simulink model "D53_LKA_Software"  (R2018b)
settings: Solver=ode3  StartTime=0.0  StopTime=10.0  FixedStep=0.01  RelTol=1e-3  EnableMultiTasking=on
model workspace (MAT data in the model file):
  MCOS : class17 (value not decoded)
  MCOS : class17 (value not decoded)
  MCOS : class17 (value not decoded)
  MCOS : class17 (value not decoded)
  MCOS : class17 (value not decoded)
  MCOS : class17 (value not decoded)
  MCOS : class17 (value not decoded)
  MCOS : class17 (value not decoded)
  MCOS : class17 (value not decoded)
  MCOS : class17 (value not decoded)
  MCOS : class17 (value not decoded)
  MCOS : class17 (value not decoded)
  MCOS : class17 (value not decoded)
  MCOS : class17 (value not decoded)
  MCOS : class17 (value not decoded)
  MCOS : class17 (value not decoded)
  MCOS : class17 (value not decoded)
  MCOS : class17 (value not decoded)
  MCOS : class17 (value not decoded)
  MCOS : class17 (value not decoded)
  MCOS : class17 (value not decoded)
  MCOS : class17 (value not decoded)
  MCOS : class17 (value not decoded)
  MCOS : class17 (value not decoded)
  MCOS : class17 (value not decoded)
  MCOS : class17 (value not decoded)
  MCOS : class17 (value not decoded)
  MCOS : class17 (value not decoded)
  MCOS : class17 (value not decoded)
  MCOS : class17 (value not decoded)
  MCOS : class17 (value not decoded)
  MCOS : class17 (value not decoded)
  MCOS : class17 (value not decoded)
  MCOS : class17 (value not decoded)
  MCOS : class17 (value not decoded)
  MCOS : class17 (value not decoded)
  MCOS : class17 (value not decoded)
  MCOS : class17 (value not decoded)
  MCOS : class17 (value not decoded)
  MCOS : class17 (value not decoded)
  MCOS : class17 (value not decoded)
  MCOS : class17 (value not decoded)
  MCOS : class17 (value not decoded)
  MCOS : class17 (value not decoded)
  MCOS : class17 (value not decoded)
  MCOS : class17 (value not decoded)
  MCOS : class17 (value not decoded)
  MCOS : class17 (value not decoded)
  MCOS : class17 (value not decoded)
  MCOS : class17 (value not decoded)
  MCOS : class17 (value not decoded)
  MCOS : class17 (value not decoded)
  MCOS : class17 (value not decoded)
  MCOS : class17 (value not decoded)
  MCOS : class17 (value not decoded)
  MCOS : class17 (value not decoded)
  MCOS : class17 (value not decoded)
  MCOS : class17 (value not decoded)
  MCOS : class17 (value not decoded)
  MCOS : class17 (value not decoded)
  MCOS : class17 (value not decoded)
  MCOS : class17 (value not decoded)
  MCOS : class17 (value not decoded)
  MCOS : class17 (value not decoded)
  MCOS : class17 (value not decoded)
  MCOS : class17 (value not decoded)
  MCOS : class17 (value not decoded)
  MCOS : class17 (value not decoded)
  MCOS : class17 (value not decoded)
  MCOS : class17 (value not decoded)
  MCOS : class17 (value not decoded)
  MCOS : class17 (value not decoded)
  MCOS : class17 (value not decoded)
  MCOS : class17 (value not decoded)
  MCOS : class17 (value not decoded)
  MCOS : class17 (value not decoded)
  MCOS : class17 (value not decoded)
  MCOS : class17 (value not decoded)
  MCOS : class17 (value not decoded)
  MCOS : class17 (value not decoded)
  MCOS : class17 (value not decoded)
  MCOS : class17 (value not decoded)
  MCOS : class17 (value not decoded)
  MCOS : class17 (value not decoded)
  MCOS : class17 (value not decoded)
  MCOS : class17 (value not decoded)
  MCOS : class17 (value not decoded)
  MCOS : class17 (value not decoded)
  MCOS : class17 (value not decoded)
undefined symbols (not defined in the file or in its folder): LKA_CarWidth, LKA_SampleTime, LKA_StrRatio_C, LKA_Veh2CamL_C, LKA_Veh2CamW_C, LKA_WhlBaseL_C, LL_CompSWA_C, LL_CrvtPrvwT_C, LL_DesDvt_C, LL_DvtComp_C, LL_DvtPrvwT_C, LL_DvtSpdDet_vDvtSpdMin_C, LL_HdAgExT_C, LL_HdAgPrvwT_C, LL_LAccMax_C, LL_LAccRMax_C, LL_LDW_EarliestWarnLine_C, LL_LDW_LatestWarnLine_C, LL_LDWS_SUPPRESS_HEADING, LL_LFClb_TFC_DiffCtlBalance, LL_LFClb_TFC_DiffCtrlMaxSWA, LL_LFClb_TFC_DiffCtrlRatio, LL_LFClb_TFC_facmGainLutGain1_C, LL_LFClb_TFC_facmGainLutGain2_C, LL_LFClb_TFC_facmIntegRatio, LL_LFClb_TFC_facmKlat_C, LL_LFClb_TFC_FfCtlRatio_C, LL_LFClb_TFC_phiIntegCtlMaxSWA_C, LL_LFClb_TFC_tiKlatPrvwT_C, LL_LFClb_TFC_vGainLutVehSpdLwr_C, LL_LFClb_TFC_vGainLutVehSpdUpr_C, LL_LKA_EarliestWarnLine_C, LL_LKA_LatestWarnLine_C, LL_LKAExPrcs_ExitC0Dvt, LL_LKAExPrcs_ExitC0Swt, LL_LKAExPrcs_tiExitTime1, LL_LKAExPrcs_tiExitTime2, LL_LKAExPrcs_tiExitTime3, LL_LKAS_OUT_OF_CONTROL_LAT_VEL, LL_LKAS_OUT_OF_CONTROL_TTLC, LL_LKASWASyn_M0, LL_LKASWASyn_M1, LL_LKASWASyn_M2, LL_LKASWASyn_M3K, LL_LKASWASyn_SWAaddMax, LL_LKASWASyn_T2, LL_LKASWASyn_tiTrqSwaRtTime, LL_LKASWASyn_tiTrqSwaTime, LL_LKASWASyn_TrqMax, LL_LKASWASyn_TrqSwaAddSwt, LL_LKASWASyn_TrqSwaRateDiff, LL_LSpdCompT_C, LL_lStpLngth_C, LL_MAX_DELAY_EPSSTAR_TIME, LL_MAX_DRIVER_TORQUE_DISABLE, LL_MAX_DRIVER_TORQUE_ENABLE, LL_MAX_LANE_WIDTH_DISABLE, LL_MAX_LANE_WIDTH_ENABLE, LL_MAX_LAT_ACC_DISABLE, LL_MAX_LAT_ACC_ENABLE ... (+30)
libraries: simulink x167, canmsglib x52, dspstat3 x3, simulink_extras x1
(part 18 of 21)

== system D53_LKA_Software/LL/LLOn/LL State Determination (LLStateDet)/LL State Machine Conditions (LLSMCon)/Disable Condition (DisblC)/Subsystem/Subsystem7 ==
  in1 : Inport
  Add : Sum
  Cast To Single : DataTypeConversion  OutDataTypeStr=uint8
  Memory : Memory  InheritSampleTime=on
  Saturation : Saturate  UpperLimit=1  LowerLimit=0
  Out1 : Outport
  wires:
  Saturation/1 -> Out1/1, Add/2
  Add/1 -> Memory/1
  Memory/1 -> Saturation/1
  in1/1 -> Cast To Single/1
  Cast To Single/1 -> Add/1

== system D53_LKA_Software/LL/LLOn/LL State Determination (LLStateDet)/LL State Machine Conditions (LLSMCon)/Disable Condition (DisblC)/Subsystem/Subsystem8 ==
  in1 : Inport
  Add : Sum
  Cast To Single : DataTypeConversion  OutDataTypeStr=uint8
  Memory : Memory  InheritSampleTime=on
  Saturation : Saturate  UpperLimit=1  LowerLimit=0
  Out1 : Outport
  wires:
  Saturation/1 -> Out1/1, Add/2
  Add/1 -> Memory/1
  Memory/1 -> Saturation/1
  in1/1 -> Cast To Single/1
  Cast To Single/1 -> Add/1

== system D53_LKA_Software/LL/LLOn/LL State Determination (LLStateDet)/LL State Machine Conditions (LLSMCon)/Disable Condition (DisblC)/Subsystem/Subsystem9 ==
  in1 : Inport
  Add : Sum
  Cast To Single : DataTypeConversion  OutDataTypeStr=uint8
  Memory : Memory  InheritSampleTime=on
  Saturation : Saturate  UpperLimit=1  LowerLimit=0
  Out1 : Outport
  wires:
  Cast To Single/1 -> Add/1
  in1/1 -> Cast To Single/1
  Memory/1 -> Saturation/1
  Add/1 -> Memory/1
  Saturation/1 -> Add/2, Out1/1

== system D53_LKA_Software/LL/LLOn/LL State Determination (LLStateDet)/LL State Machine Conditions (LLSMCon)/Disable Condition (DisblC)/Vehicle State Condition (VehStateC)/Emergency Light Enable Condition (EmgcyLghtEC) ==
  EmgcyLghtEC_bsStLampState : Inport
  Add : Sum
  Bus Selector : BusSelector  OutputSignals=BCM_Double_Light,BCM_Left_Light,BCM_Right_Light
  Compare To Constant{,1..3} (4 alike) : simulink/Logic and Bit Operations/Compare To Constant  relop=>  const=0  OutDataTypeStr=boolean
  Constant : Constant  Value=3  OutDataTypeStr=single
  Constant1 : Constant  Value=-1  OutDataTypeStr=single
  Logical Operator : Logic  Operator=OR  Inputs=3  AllPortsSameDT=off  OutDataTypeStr=boolean
  Memory : Memory  InheritSampleTime=on
  Saturation : Saturate  UpperLimit=200  LowerLimit=-1
  Switch : Switch  Criteria=u2 > Threshold
  EmgcyLghtEC_stEmgcyLghtECFlg : Outport
  wires:
  Compare To Constant2/1 -> Logical Operator/2
  Compare To Constant1/1 -> Logical Operator/1
  EmgcyLghtEC_bsStLampState/1 -> Bus Selector/1
  Bus Selector/1 -> Compare To Constant1/1  "<BCM_Double_Light>"
  Bus Selector/2 -> Compare To Constant2/1  "<BCM_Left_Light>"
  Logical Operator/1 -> Switch/2
  Constant/1 -> Switch/1
  Constant1/1 -> Switch/3
  Switch/1 -> Add/1
  Add/1 -> Saturation/1
  Saturation/1 -> Compare To Constant/1, Memory/1
  Memory/1 -> Add/2
  Compare To Constant/1 -> EmgcyLghtEC_stEmgcyLghtECFlg/1
  Bus Selector/3 -> Compare To Constant3/1  "<BCM_Right_Light>"
  Compare To Constant3/1 -> Logical Operator/3

== system D53_LKA_Software/LL/LLOn/LL State Determination (LLStateDet)/LL State Machine Conditions (LLSMCon)/Disable Condition (DisblC)/Vehicle State Condition (VehStateC)/Gear Disable Condition (GearDC) ==
  In1 : Inport
  Compare To Constant : simulink/Logic and Bit Operations/Compare To Constant  relop=~=  const=3  OutDataTypeStr=boolean
  GearDC_stGearDCFlg : Outport
  wires:
  In1/1 -> Compare To Constant/1
  Compare To Constant/1 -> GearDC_stGearDCFlg/1

== system D53_LKA_Software/LL/LLOn/LL State Determination (LLStateDet)/LL State Machine Conditions (LLSMCon)/Disable Condition (DisblC)/Vehicle State Condition (VehStateC)/Vehicle Speed Disable Condition (VehSpdDC) ==
  VehSpdDC_stDACMode : Inport
  VehSpdDC_vVehSpd : Inport  Port=2
  VehSpdDC_vLDWVehSpdMax_C : Inport  Port=3
  VehSpdDC_vLKAVehSpdMax_C : Inport  Port=4
  VehSpdDC_vVehSpdMin_C : Inport  Port=5
  Interval Test Dynamic : simulink/Logic and Bit Operations/Interval Test Dynamic  IntervalClosedRight=off  IntervalClosedLeft=off  OutDataTypeStr=boolean
      settings: SourceProductName=Simulink  SourceProductBaseCode=SL
  Logical Operator : Logic  Operator=NOT  AllPortsSameDT=off  OutDataTypeStr=boolean
  Switch : Switch  Threshold=2
  VehSpdDC_stVehSpdDCFlg : Outport
  wires:
  Interval Test Dynamic/1 -> Logical Operator/1
  VehSpdDC_vVehSpd/1 -> Interval Test Dynamic/2
  VehSpdDC_vVehSpdMin_C/1 -> Interval Test Dynamic/3
  Logical Operator/1 -> VehSpdDC_stVehSpdDCFlg/1
  VehSpdDC_stDACMode/1 -> Switch/2
  VehSpdDC_vLKAVehSpdMax_C/1 -> Switch/1
  Switch/1 -> Interval Test Dynamic/1
  VehSpdDC_vLDWVehSpdMax_C/1 -> Switch/3

== system D53_LKA_Software/LL/LLOn/LL State Determination (LLStateDet)/LL State Machine Conditions (LLSMCon)/Disable Condition (DisblC)/Vehicle State Condition (VehStateC)/Vehicle State Condition Synthesis (VehStateCSyn) ==
  VehStateCSyn_stVehSpdDCFlg : Inport
  VehStateCSyn_stEmgcyLghtDCFlg : Inport  Port=2
  VehStateCSyn_stGearDCFlg : Inport  Port=3
  Logical Operator3 : Logic  Operator=OR  Inputs=3  AllPortsSameDT=off  OutDataTypeStr=boolean
  VehStateCSyn_stVehStateCSyn : Outport
  wires:
  VehStateCSyn_stVehSpdDCFlg/1 -> Logical Operator3/1
  VehStateCSyn_stGearDCFlg/1 -> Logical Operator3/3
  Logical Operator3/1 -> VehStateCSyn_stVehStateCSyn/1
  VehStateCSyn_stEmgcyLghtDCFlg/1 -> Logical Operator3/2

== system D53_LKA_Software/LL/LLOn/LL State Determination (LLStateDet)/LL State Machine Conditions (LLSMCon)/Enable Condition (EnaC)/Enable Condition Synthesis (EnaCSyn)/If Action Subsystem ==
  Action Port : ActionPort  InitializeStates=reset
  Constant : Constant  OutDataTypeStr=boolean  SampleTime=-1
  Out : Outport
  wires:
  Constant/1 -> Out/1

== system D53_LKA_Software/LL/LLOn/LL State Determination (LLStateDet)/LL State Machine Conditions (LLSMCon)/Enable Condition (EnaC)/Enable Condition Synthesis (EnaCSyn)/If Action Subsystem2 ==
  Action Port : ActionPort  InitializeStates=reset
  Constant : Constant  OutDataTypeStr=boolean  SampleTime=-1
  Out : Outport
  wires:
  Constant/1 -> Out/1

== system D53_LKA_Software/LL/LLOn/LL State Determination (LLStateDet)/LL State Machine Conditions (LLSMCon)/Enable Condition (EnaC)/Enable Condition Synthesis (EnaCSyn)/If Action Subsystem3 ==
  Action Port : ActionPort  InitializeStates=reset
  Constant : Constant  Value=0  OutDataTypeStr=boolean
  Out : Outport
  wires:
  Constant/1 -> Out/1

== system D53_LKA_Software/LL/LLOn/LL State Determination (LLStateDet)/LL State Machine Conditions (LLSMCon)/Enable Condition (EnaC)/Enable Condition Synthesis (EnaCSyn)/If Action Subsystem4 ==
  Action Port : ActionPort  InitializeStates=reset
  Constant : Constant  Value=0  OutDataTypeStr=boolean
  Out : Outport
  wires:
  Constant/1 -> Out/1

== system D53_LKA_Software/LL/LLOn/LL State Determination (LLStateDet)/LL State Machine Conditions (LLSMCon)/Enable Condition (EnaC)/LDW Own Condition (LDWOwnC)/LDW Own Condition Synthesis (LDWOwnCSyn) ==
  LDWOwnCSyn_stDACMode : Inport
  LDWOwnCSyn_stVehPosChk : Inport  Port=2
  Compare To Constant : simulink/Logic and Bit Operations/Compare To Constant  relop=>=  const=1  OutDataTypeStr=boolean
  Compare To Constant1 : simulink/Logic and Bit Operations/Compare To Constant  relop===  const=1  OutDataTypeStr=boolean
  Logical Operator : Logic  AllPortsSameDT=off  OutDataTypeStr=boolean
  LDWOwnCSyn_stLDWOwnCSyn : Outport
  wires:
  LDWOwnCSyn_stDACMode/1 -> Compare To Constant/1
  LDWOwnCSyn_stVehPosChk/1 -> Compare To Constant1/1
  Compare To Constant/1 -> Logical Operator/1
  Compare To Constant1/1 -> Logical Operator/2
  Logical Operator/1 -> LDWOwnCSyn_stLDWOwnCSyn/1

== system D53_LKA_Software/LL/LLOn/LL State Determination (LLStateDet)/LL State Machine Conditions (LLSMCon)/Enable Condition (EnaC)/LDW Own Condition (LDWOwnC)/Vehicle Position Check (VehPosChk) ==
  VehPosChk_LaneWidth : Inport
  VehPosChk_bsDvtInfo : Inport  Port=2
  VehPosChk_lWarnLine_C : Inport  Port=3
  Bus Selector : BusSelector  OutputSignals=ILftDvt,IRgtDvt
  Logical Operator : Logic  AllPortsSameDT=off  OutDataTypeStr=boolean
  Relational Operator1 : RelationalOperator  OutDataTypeStr=boolean  RndMeth=Nearest
  Relational Operator2 : RelationalOperator  OutDataTypeStr=boolean  RndMeth=Nearest
  Subsystem : Subsystem
  VehPosChk_stVehPosChk : Outport
  wires:
  Bus Selector/1 -> Relational Operator1/1  "<ILftDvt>"
  Bus Selector/2 -> Relational Operator2/1  "<IRgtDvt>"
  Relational Operator1/1 -> Logical Operator/1
  Relational Operator2/1 -> Logical Operator/2
  Logical Operator/1 -> VehPosChk_stVehPosChk/1
  VehPosChk_bsDvtInfo/1 -> Bus Selector/1
  Subsystem/1(EnableLine) -> Relational Operator1/2, Relational Operator2/2
  VehPosChk_lWarnLine_C/1 -> Subsystem/1(WarnLine_C)
  VehPosChk_LaneWidth/1 -> Subsystem/2(LaneWidth)

== system D53_LKA_Software/LL/LLOn/LL State Determination (LLStateDet)/LL State Machine Conditions (LLSMCon)/Enable Condition (EnaC)/LKA Own Condition (LKAOwnC)/EPS State Condition (EPSStC) ==
  EPSStC_bsEPSInfo : Inport
  Bus Selector : BusSelector  OutputSignals=EPS_LKA_State
  Compare To Constant1 : simulink/Logic and Bit Operations/Compare To Constant  relop===  const=2  OutDataTypeStr=boolean
  Compare To Constant2 : simulink/Logic and Bit Operations/Compare To Constant  relop===  const=1  OutDataTypeStr=boolean
  Logical Operator : Logic  Operator=OR  AllPortsSameDT=off  OutDataTypeStr=boolean
  EPSStC_tfEPSCtlEC : Outport
  wires:
  EPSStC_bsEPSInfo/1 -> Bus Selector/1
  Logical Operator/1 -> EPSStC_tfEPSCtlEC/1
  Bus Selector/1 -> Compare To Constant2/1, Compare To Constant1/1  "<EPS_LKA_State>"
  Compare To Constant1/1 -> Logical Operator/1
  Compare To Constant2/1 -> Logical Operator/2

== system D53_LKA_Software/LL/LLOn/LL State Determination (LLStateDet)/LL State Machine Conditions (LLSMCon)/Enable Condition (EnaC)/LKA Own Condition (LKAOwnC)/Exit Lane Delay (ExLaneDel) ==
  ExLaneDel_stVehExLane : Inport
  ExLaneDel_tiExLaneDelT : Inport  Port=2
  Bus Selector2 : BusSelector  OutputSignals=LKA_SampleTime
  Cast To Single1 : DataTypeConversion  OutDataTypeStr=uint16
  Compare To Zero : simulink/Logic and Bit Operations/Compare To Zero  relop===  OutDataTypeStr=boolean
  Detect Fall Nonpositive : simulink/Logic and Bit Operations/Detect Fall Nonpositive  vinit=0  OutDataTypeStr=boolean
      settings: SourceProductName=Simulink  SourceProductBaseCode=SL
  Detect Rise Positive1 : simulink/Logic and Bit Operations/Detect Rise Positive  vinit=0  OutDataTypeStr=boolean
  Divide : Product  Inputs=*/
  If Action Subsystem3 : Subsystem  TreatAsAtomicUnit=on
  If Action Subsystem4 : Subsystem  TreatAsAtomicUnit=on
  If Action Subsystem5 : Subsystem  TreatAsAtomicUnit=on
  If1 : If  NumInputs=4  IfExpression=u1 == 1 & u2 == 1  ElseIfExpressions=u3 == 0 & u4 == 1
  Memory1 : Memory  InheritSampleTime=on
  Memory2 : Memory  InheritSampleTime=on
  Merge : Merge  Inputs=3
  Sum Condition1 : Subsystem  TreatAsAtomicUnit=on
  ExLaneDel_stExLaneDel : Outport
  wires:
  Merge/1 -> Memory1/1, Sum Condition1/1(In), Sum Condition1/Enable, Compare To Zero/1
  Memory1/1 -> If Action Subsystem5/1(In1)
  Memory2/1 -> Detect Fall Nonpositive/1, If1/3
  ExLaneDel_tiExLaneDelT/1 -> Divide/1
  If1/2 -> If Action Subsystem4/Action
  If1/1 -> If Action Subsystem3/Action
  If1/3 -> If Action Subsystem5/Action
  Detect Rise Positive1/1 -> If1/2
  ExLaneDel_stVehExLane/1 -> If1/1, Detect Rise Positive1/1
  Detect Fall Nonpositive/1 -> If1/4
  If Action Subsystem3/1(Out) -> Merge/1
  If Action Subsystem5/1(Out) -> Merge/3
  If Action Subsystem4/1(Out) -> Merge/2
  Sum Condition1/1(Out) -> Memory2/1
  Compare To Zero/1 -> ExLaneDel_stExLaneDel/1
  Divide/1 -> Cast To Single1/1
  Bus Selector2/1 -> Divide/2  "<LKA_SampleTime>"
  [LLClb_bsConstantClb] -> Bus Selector2/1
  Cast To Single1/1 -> Sum Condition1/2(Sum)

== system D53_LKA_Software/LL/LLOn/LL State Determination (LLStateDet)/LL State Machine Conditions (LLSMCon)/Enable Condition (EnaC)/LKA Own Condition (LKAOwnC)/LKA Own Condition Synthesis (LKAOwnCSyn) ==
  LKAOwnCSyn_stDACMode : Inport
  LKAOwnCSyn_stEPSCtlEC : Inport  Port=2
  LKAOwnCSyn_stVehLSpdC : Inport  Port=3
  LKAOwnCSyn_stVehPosChk : Inport  Port=4
  LKAOwnCSyn_stExLaneDel : Inport  Port=5
  Compare To Constant : simulink/Logic and Bit Operations/Compare To Constant  relop===  const=2  OutDataTypeStr=boolean
  Compare To Constant{1..2,4..5} (4 alike) : simulink/Logic and Bit Operations/Compare To Constant  relop===  const=1  OutDataTypeStr=boolean
  Logical Operator : Logic  Inputs=4  AllPortsSameDT=off  OutDataTypeStr=boolean
  LKAOwnCSyn_stLKAPptyCSyn : Outport
  wires:
  LKAOwnCSyn_stDACMode/1 -> Compare To Constant/1
  LKAOwnCSyn_stVehPosChk/1 -> Compare To Constant1/1
  Logical Operator/1 -> LKAOwnCSyn_stLKAPptyCSyn/1
  LKAOwnCSyn_stEPSCtlEC/1 -> Compare To Constant2/1
  LKAOwnCSyn_stExLaneDel/1 -> Compare To Constant5/1
  Compare To Constant/1 -> Logical Operator/1
  Compare To Constant2/1 -> Logical Operator/2
  Compare To Constant4/1 -> Logical Operator/3
  Compare To Constant1/1 -> Logical Operator/4
  Compare To Constant5/1 -> ?
  LKAOwnCSyn_stVehLSpdC/1 -> Compare To Constant4/1

== system D53_LKA_Software/LL/LLOn/LL State Determination (LLStateDet)/LL State Machine Conditions (LLSMCon)/Enable Condition (EnaC)/LKA Own Condition (LKAOwnC)/Vehicle Lateral Speed Condition (VehLSpdC) ==
  VehLSpdC_bsTTLCInfo : Inport
  VehLSpdC_vVehLSpdMax_C : Inport  Port=2
  Abs1 : Abs
  Abs2 : Abs
  Bus Selector2 : BusSelector  OutputSignals=vLft,vRgt
  Logical Operator : Logic  AllPortsSameDT=off  OutDataTypeStr=boolean
  Relational Operator2 : RelationalOperator  Operator=<=  OutDataTypeStr=boolean  RndMeth=Nearest
  Relational Operator3 : RelationalOperator  Operator=<=  OutDataTypeStr=boolean  RndMeth=Nearest
  VehLSpdC_stVehLSpdC : Outport
  wires:
  VehLSpdC_vVehLSpdMax_C/1 -> Relational Operator3/2, Relational Operator2/2
  Abs1/1 -> Relational Operator2/1
  Relational Operator2/1 -> Logical Operator/1
  Abs2/1 -> Relational Operator3/1
  Bus Selector2/1 -> Abs1/1  "<vLft>"
  Bus Selector2/2 -> Abs2/1  "<vRgt>"
  VehLSpdC_bsTTLCInfo/1 -> Bus Selector2/1
  Logical Operator/1 -> VehLSpdC_stVehLSpdC/1
  Relational Operator3/1 -> Logical Operator/2

== system D53_LKA_Software/LL/LLOn/LL State Determination (LLStateDet)/LL State Machine Conditions (LLSMCon)/Enable Condition (EnaC)/LKA Own Condition (LKAOwnC)/Vehicle Position Check (VehPosChk)1 ==
  VehPosChk_LaneWidth : Inport
  VehPosChk_bsDvtInfo : Inport  Port=2
  VehPosChk_lWarnLineMax_C : Inport  Port=3
  VehPosChk_lWarnLineMin_C : Inport  Port=4
  Bus Selector : BusSelector  OutputSignals=ILftDvt,IRgtDvt
  Logical Operator : Logic  AllPortsSameDT=off  OutDataTypeStr=boolean
  Logical Operator1 : Logic  Operator=OR  AllPortsSameDT=off  OutDataTypeStr=boolean
  Relational Operator1 : RelationalOperator  OutDataTypeStr=boolean  RndMeth=Nearest
  Relational Operator2 : RelationalOperator  OutDataTypeStr=boolean  RndMeth=Nearest
  Relational Operator3 : RelationalOperator  Operator=<=  OutDataTypeStr=boolean  RndMeth=Nearest
  Relational Operator4 : RelationalOperator  Operator=<=  OutDataTypeStr=boolean  RndMeth=Nearest
  Subsystem : Subsystem
  VehPosChk_stVehPosChk : Outport
  VehPosChk_stVehExLane : Outport  Port=2
  wires:
  Bus Selector/1 -> Relational Operator4/1, Relational Operator1/1  "<ILftDvt>"
  Bus Selector/2 -> Relational Operator2/1, Relational Operator3/1  "<IRgtDvt>"
  Relational Operator1/1 -> Logical Operator/1
  Relational Operator2/1 -> Logical Operator/2
  Logical Operator/1 -> VehPosChk_stVehPosChk/1
  VehPosChk_bsDvtInfo/1 -> Bus Selector/1
  Subsystem/1(EnableLine) -> Relational Operator1/2, Relational Operator2/2
  VehPosChk_lWarnLineMax_C/1 -> Subsystem/1(WarnLine_C)
  VehPosChk_LaneWidth/1 -> Subsystem/2(LaneWidth)
  Logical Operator1/1 -> VehPosChk_stVehExLane/1
  Relational Operator3/1 -> Logical Operator1/2
  VehPosChk_lWarnLineMin_C/1 -> Relational Operator3/2, Relational Operator4/2
  Relational Operator4/1 -> Logical Operator1/1

== system D53_LKA_Software/LL/LLOn/LL State Determination (LLStateDet)/LL State Machine Conditions (LLSMCon)/Enable Condition (EnaC)/Lane Condition (LaneC)/Lane C1 Detection (LaneC1Det) ==
  LaneWDet_facmL0C1 : Inport
  LaneWDet_facmR0C1 : Inport  Port=2
  Abs : Abs
  Add : Sum  Inputs=+-  OutDataTypeStr=single
  Compare To Constant1 : simulink/Logic and Bit Operations/Compare To Constant  relop=<=  const=0.025  OutDataTypeStr=boolean
  LaneC1Det_stLaneC1DetFlg : Outport
  wires:
  LaneWDet_facmR0C1/1 -> Add/2
  LaneWDet_facmL0C1/1 -> Add/1
  Add/1 -> Abs/1
  Compare To Constant1/1 -> LaneC1Det_stLaneC1DetFlg/1
  Abs/1 -> Compare To Constant1/1

== system D53_LKA_Software/LL/LLOn/LL State Determination (LLStateDet)/LL State Machine Conditions (LLSMCon)/Enable Condition (EnaC)/Lane Condition (LaneC)/Lane Condition Synthesis (LaneCSyn) ==
  LaneCSyn_stLaneQlECFlg : Inport
  LaneCSyn_stLaneWDetFlg : Inport  Port=2
  LaneCSyn_stLaneCrvtDetFlg : Inport  Port=3
  LaneCSyn_stLaneC1DetFlg : Inport  Port=4
  Logical Operator3 : Logic  Inputs=4  AllPortsSameDT=off  OutDataTypeStr=boolean
  LaneCSyn_stLaneCSyn : Outport
  wires:
  LaneCSyn_stLaneQlECFlg/1 -> Logical Operator3/1
  LaneCSyn_stLaneCrvtDetFlg/1 -> Logical Operator3/3
  Logical Operator3/1 -> LaneCSyn_stLaneCSyn/1
  LaneCSyn_stLaneWDetFlg/1 -> Logical Operator3/2
  LaneCSyn_stLaneC1DetFlg/1 -> Logical Operator3/4

== system D53_LKA_Software/LL/LLOn/LL State Determination (LLStateDet)/LL State Machine Conditions (LLSMCon)/Enable Condition (EnaC)/Lane Condition (LaneC)/Lane Curvature Detection (LaneCrvtDet) ==
  LaneCrvtDet_crPrvwCrvt : Inport
  LaneCrvtDet_crLaneCrvtMax_C : Inport  Port=2
  Abs : Abs
  Constant : Constant  Value=0  OutDataTypeStr=single  SampleTime=-1
  Interval Test Dynamic : simulink/Logic and Bit Operations/Interval Test Dynamic  IntervalClosedRight=on  IntervalClosedLeft=on  OutDataTypeStr=boolean
      settings: SourceProductName=Simulink  SourceProductBaseCode=SL
  LaneCrvtDet_stLaneCrvtDetFlg : Outport
  wires:
  Interval Test Dynamic/1 -> LaneCrvtDet_stLaneCrvtDetFlg/1
  LaneCrvtDet_crLaneCrvtMax_C/1 -> Interval Test Dynamic/1
  Constant/1 -> Interval Test Dynamic/3
  LaneCrvtDet_crPrvwCrvt/1 -> Abs/1
  Abs/1 -> Interval Test Dynamic/2

== system D53_LKA_Software/LL/LLOn/LL State Determination (LLStateDet)/LL State Machine Conditions (LLSMCon)/Enable Condition (EnaC)/Lane Condition (LaneC)/Lane Quality Enable Condition (LaneQlEC) ==
  LaneQlEC_stFacmL0Ql : Inport
  LaneQlEC_stFacmR0Ql : Inport  Port=2
  Compare To Constant : simulink/Logic and Bit Operations/Compare To Constant  relop=>  const=2  OutDataTypeStr=boolean
  Compare To Constant1 : simulink/Logic and Bit Operations/Compare To Constant  relop=>  const=2  OutDataTypeStr=boolean
  Logical Operator : Logic  AllPortsSameDT=off  OutDataTypeStr=boolean
  LaneQlEC_stLaneQlECFlg : Outport
  wires:
  LaneQlEC_stFacmL0Ql/1 -> Compare To Constant/1
  LaneQlEC_stFacmR0Ql/1 -> Compare To Constant1/1
  Compare To Constant/1 -> Logical Operator/1
  Compare To Constant1/1 -> Logical Operator/2
  Logical Operator/1 -> LaneQlEC_stLaneQlECFlg/1

== system D53_LKA_Software/LL/LLOn/LL State Determination (LLStateDet)/LL State Machine Conditions (LLSMCon)/Enable Condition (EnaC)/Lane Condition (LaneC)/Lane Width Detection (LaneWDet) ==
  LaneWDet_LaneWidth : Inport
  LaneWDet_lLaneWMax : Inport  Port=2
  LaneWDet_lLaneWMin : Inport  Port=3
  Abs1 : Abs
  Interval Test Dynamic : simulink/Logic and Bit Operations/Interval Test Dynamic  IntervalClosedRight=on  IntervalClosedLeft=on  OutDataTypeStr=boolean
      settings: SourceProductName=Simulink  SourceProductBaseCode=SL
  LaneWDet_stLaneWDetFlg : Outport
  wires:
  Interval Test Dynamic/1 -> LaneWDet_stLaneWDetFlg/1
  LaneWDet_lLaneWMax/1 -> Interval Test Dynamic/1
  LaneWDet_lLaneWMin/1 -> Interval Test Dynamic/3
  Abs1/1 -> Interval Test Dynamic/2
  LaneWDet_LaneWidth/1 -> Abs1/1

== system D53_LKA_Software/LL/LLOn/LL State Determination (LLStateDet)/LL State Machine Conditions (LLSMCon)/Enable Condition (EnaC)/Vehicle State Condition (VehStateC)/Emergency Light Enable Condition (EmgcyLghtEC) ==
  EmgcyLghtEC_bsStLampState : Inport
  Add : Sum
  Bus Selector : BusSelector  OutputSignals=BCM_Double_Light,BCM_Left_Light,BCM_Right_Light
  Compare To Constant : simulink/Logic and Bit Operations/Compare To Constant  relop=<=  const=0  OutDataTypeStr=boolean
  Compare To Constant1 : simulink/Logic and Bit Operations/Compare To Constant  relop=>  const=0  OutDataTypeStr=boolean
  Compare To Constant2 : simulink/Logic and Bit Operations/Compare To Constant  relop=>  const=0  OutDataTypeStr=boolean
  Compare To Constant3 : simulink/Logic and Bit Operations/Compare To Constant  relop=>  const=0  OutDataTypeStr=boolean
  Constant : Constant  Value=3  OutDataTypeStr=single
  Constant1 : Constant  Value=-1  OutDataTypeStr=single
  Logical Operator : Logic  Operator=OR  Inputs=3  AllPortsSameDT=off  OutDataTypeStr=boolean
  Memory : Memory  InheritSampleTime=on
  Saturation : Saturate  UpperLimit=200  LowerLimit=-1
  Switch : Switch  Criteria=u2 > Threshold
  EmgcyLghtEC_stEmgcyLghtECFlg : Outport
  wires:
  Compare To Constant2/1 -> Logical Operator/2
  Compare To Constant1/1 -> Logical Operator/1
  EmgcyLghtEC_bsStLampState/1 -> Bus Selector/1
  Bus Selector/1 -> Compare To Constant1/1  "<BCM_Double_Light>"
  Bus Selector/2 -> Compare To Constant2/1  "<BCM_Left_Light>"
  Logical Operator/1 -> Switch/2
  Constant/1 -> Switch/1
  Constant1/1 -> Switch/3
  Switch/1 -> Add/1
  Add/1 -> Saturation/1
  Saturation/1 -> Compare To Constant/1, Memory/1
  Memory/1 -> Add/2
  Compare To Constant/1 -> EmgcyLghtEC_stEmgcyLghtECFlg/1
  Bus Selector/3 -> Compare To Constant3/1  "<BCM_Right_Light>"
  Compare To Constant3/1 -> Logical Operator/3

== system D53_LKA_Software/LL/LLOn/LL State Determination (LLStateDet)/LL State Machine Conditions (LLSMCon)/Enable Condition (EnaC)/Vehicle State Condition (VehStateC)/Gear Enable Condition (GearEC) ==
  GearEC_bsTCUState : Inport
  Bus Selector : BusSelector  OutputSignals=TCU_ActualGear
  Compare To Constant : simulink/Logic and Bit Operations/Compare To Constant  relop===  const=3  OutDataTypeStr=boolean
  GearEC_stGearECFlg : Outport
  wires:
  GearEC_bsTCUState/1 -> Bus Selector/1
  Bus Selector/1 -> Compare To Constant/1  "<TCU_ActualGear>"
  Compare To Constant/1 -> GearEC_stGearECFlg/1

== system D53_LKA_Software/LL/LLOn/LL State Determination (LLStateDet)/LL State Machine Conditions (LLSMCon)/Enable Condition (EnaC)/Vehicle State Condition (VehStateC)/Vehicle Speed Enable Condition (VehSpdEC) ==
  VehSpdEC_stDACMode : Inport
  VehSpdEC_vVehSpd : Inport  Port=2
  VehSpdEC_vLDWVehSpdMax_C : Inport  Port=3
  VehSpdEC_vLKAVehSpdMax_C : Inport  Port=4
  VehSpdEC_vVehSpdMin_C : Inport  Port=5
  Interval Test Dynamic : simulink/Logic and Bit Operations/Interval Test Dynamic  IntervalClosedRight=on  IntervalClosedLeft=on  OutDataTypeStr=boolean
      settings: SourceProductName=Simulink  SourceProductBaseCode=SL
  Switch : Switch  Threshold=2
  VehSpdEC_stVehSpdECFlg : Outport
  wires:
  VehSpdEC_vVehSpd/1 -> Interval Test Dynamic/2
  VehSpdEC_vVehSpdMin_C/1 -> Interval Test Dynamic/3
  Interval Test Dynamic/1 -> VehSpdEC_stVehSpdECFlg/1
  VehSpdEC_stDACMode/1 -> Switch/2
  VehSpdEC_vLKAVehSpdMax_C/1 -> Switch/1
  Switch/1 -> Interval Test Dynamic/1
  VehSpdEC_vLDWVehSpdMax_C/1 -> Switch/3

== system D53_LKA_Software/LL/LLOn/LL State Determination (LLStateDet)/LL State Machine Conditions (LLSMCon)/Enable Condition (EnaC)/Vehicle State Condition (VehStateC)/Vehicle State Condition Synthesis (VehStateCSyn) ==
  VehStateCSyn_stVehSpdECFlg : Inport
  VehStateCSyn_stEmgcyLghtECFlg : Inport  Port=2
  VehStateCSyn_stGearECFlg : Inport  Port=3
  Logical Operator : Logic  Inputs=3  AllPortsSameDT=off  OutDataTypeStr=boolean
  VehStateCSyn_stVehStateCSyn : Outport
  wires:
  VehStateCSyn_stVehSpdECFlg/1 -> Logical Operator/1
  VehStateCSyn_stGearECFlg/1 -> Logical Operator/3
  Logical Operator/1 -> VehStateCSyn_stVehStateCSyn/1
  VehStateCSyn_stEmgcyLghtECFlg/1 -> Logical Operator/2

== system D53_LKA_Software/SignalBusCreator/Body Electric System State Receive and Processing (BESRx)/Steering Lamp CAN Frame PreProcess (StLampCANFrmPPrcs)/CAN Diagnosis (CANDia)/CheckSum Diagnosis (ChkSumDia)/Bit Check(BChk)/Bit Operating (BOp) ==
  note: Checksum Preprocess -- ChksumPre
  note: CheckSum Error Flag Discription:
      | 1 : Fault
      | 0 : Normal
  BOp_bByte0 : Inport
  BOp_bByte1 : Inport  Port=2
  BOp_bByte2 : Inport  Port=3
  BOp_bByte3 : Inport  Port=4
  BOp_bByte4 : Inport  Port=5
  BOp_bByte5 : Inport  Port=6
  BOp_bByte6 : Inport  Port=7
  BOp_bByte7 : Inport  Port=8
  Add : Sum  Inputs=+++++++
  Add1 : Sum  Inputs=+-
  Add2 : Sum  Inputs=+-
  ChksumPre1 : Subsystem
  ChksumPre2 : Subsystem
  ChksumPre3 : Subsystem
  ChksumPre4 : Subsystem
  ChksumPre5 : Subsystem
  ChksumPre6 : Subsystem
  ChksumPre7 : Subsystem
  Constant : Constant  Value=256  OutDataTypeStr=uint16  SampleTime=-1
  Constant1 : Constant  Value=255  OutDataTypeStr=uint8  SampleTime=-1
  Constant2 : Constant  OutDataTypeStr=uint8  SampleTime=-1
  Constant3 : Constant  Value=0  OutDataTypeStr=uint8  SampleTime=-1
  Data Type Conversion6 : DataTypeConversion  OutDataTypeStr=uint8
  Math Function : Math  Operator=mod  OutputSignalType=real  SaturateOnIntegerOverflow=on
  Switch : Switch  Criteria=u2 ~= 0
  BOp_efChkSumErrFlg : Outport
  wires:
  Add2/1 -> Switch/2
  Add1/1 -> Add2/2
  BOp_bByte0/1 -> Add2/1
  ChksumPre3/1(Out1) -> Add/3
  ChksumPre2/1(Out1) -> Add/2
  Data Type Conversion6/1 -> Add1/2
  Add/1 -> Math Function/1
  Constant/1 -> Math Function/2
  Math Function/1 -> Data Type Conversion6/1
  Constant1/1 -> Add1/1
  BOp_bByte1/1 -> ChksumPre1/1(In1)
  ChksumPre1/1(Out1) -> Add/1
  BOp_bByte2/1 -> ChksumPre2/1(In1), ChksumPre3/1(In1), ChksumPre4/1(In1)
  ChksumPre4/1(Out1) -> Add/4
  BOp_bByte3/1 -> ChksumPre5/1(In1)
  BOp_bByte4/1 -> ChksumPre5/2(In2)
  ChksumPre5/1(Out1) -> Add/5
  BOp_bByte5/1 -> ChksumPre6/1(In1)
  BOp_bByte6/1 -> ChksumPre6/2(In2)
  ChksumPre6/1(Out1) -> Add/6
  ChksumPre7/1(Out1) -> Add/7
  BOp_bByte7/1 -> ChksumPre7/1(In1)
  Constant2/1 -> Switch/1
  Constant3/1 -> Switch/3
  Switch/1 -> BOp_efChkSumErrFlg/1

== system D53_LKA_Software/SignalBusCreator/Function Keys State Receive and Processing (FKeyStRx)/Key Enable CAN Frame PreProcess (KeyEnaCANFrmPPrcs)/CAN Diagnosis (CANDia)/CheckSum Diagnosis (ChkSumDia)/Bit Check(BChk)/Bit Operating (BOp) ==
  note: CheckSum Error Flag Discription:
      | 1 : Fault
      | 0 : Normal
  note: Checksum Preprocess -- ChksumPre
  BOp_bByte0 : Inport
  BOp_bByte1 : Inport  Port=2
  BOp_bByte2 : Inport  Port=3
  BOp_bByte3 : Inport  Port=4
  BOp_bByte4 : Inport  Port=5
  BOp_bByte5 : Inport  Port=6
  BOp_bByte6 : Inport  Port=7
  BOp_bByte7 : Inport  Port=8
  Add : Sum  Inputs=+++++++
  Add1 : Sum  Inputs=+-
  Add2 : Sum  Inputs=+-
  ChksumPre1 : Subsystem
  ChksumPre2 : Subsystem
  ChksumPre3 : Subsystem
  ChksumPre4 : Subsystem
  ChksumPre5 : Subsystem
  ChksumPre6 : Subsystem
  ChksumPre7 : Subsystem
  Constant : Constant  Value=256  OutDataTypeStr=uint16  SampleTime=-1
  Constant1 : Constant  Value=255  OutDataTypeStr=uint8  SampleTime=-1
  Constant2 : Constant  OutDataTypeStr=uint8  SampleTime=-1
  Constant3 : Constant  Value=0  OutDataTypeStr=uint8  SampleTime=-1
  Data Type Conversion6 : DataTypeConversion  OutDataTypeStr=uint8
  Math Function : Math  Operator=mod  OutputSignalType=real  SaturateOnIntegerOverflow=on
  Switch : Switch  Criteria=u2 ~= 0
  BOp_efChkSumErrFlg : Outport
  wires:
  Switch/1 -> BOp_efChkSumErrFlg/1
  Constant3/1 -> Switch/3
  Constant2/1 -> Switch/1
  BOp_bByte7/1 -> ChksumPre7/1(In1)
  ChksumPre7/1(Out1) -> Add/7
  ChksumPre6/1(Out1) -> Add/6
  BOp_bByte6/1 -> ChksumPre6/2(In2)
  BOp_bByte5/1 -> ChksumPre6/1(In1)
  ChksumPre5/1(Out1) -> Add/5
  BOp_bByte4/1 -> ChksumPre5/2(In2)
  BOp_bByte3/1 -> ChksumPre5/1(In1)
  ChksumPre4/1(Out1) -> Add/4
  BOp_bByte2/1 -> ChksumPre4/1(In1), ChksumPre3/1(In1), ChksumPre2/1(In1)
  ChksumPre1/1(Out1) -> Add/1
  BOp_bByte1/1 -> ChksumPre1/1(In1)
  Constant1/1 -> Add1/1
  Math Function/1 -> Data Type Conversion6/1
  Constant/1 -> Math Function/2
  Add/1 -> Math Function/1
  Data Type Conversion6/1 -> Add1/2
  ChksumPre2/1(Out1) -> Add/2
  ChksumPre3/1(Out1) -> Add/3
  BOp_bByte0/1 -> Add2/1
  Add1/1 -> Add2/2
  Add2/1 -> Switch/2

== system D53_LKA_Software/SignalBusCreator/Lanes Information Receive and Processing (LaneRx)/L0 Information (L0Info) /CAN Diagnosis (CANDia)/CheckSum Diagnosis (ChkSumDia)/Bit Check(BChk)/Bit Operating (BOp) ==
  note: Checksum Preprocess -- ChksumPre
  note: CheckSum Error Flag Discription:
      | 1 : Fault
      | 0 : Normal
  Chksum in Frame : Inport
  BOp_bByte1 : Inport  Port=2
  BOp_bByte2 : Inport  Port=3
  BOp_bByte3 : Inport  Port=4
  BOp_bByte4 : Inport  Port=5
  BOp_bByte5 : Inport  Port=6
  BOp_bByte6 : Inport  Port=7
  BOp_bByte7 : Inport  Port=8
  Add : Sum  Inputs=+++++++
  Add1 : Sum  Inputs=+-
  Add2 : Sum  Inputs=+-
  ChksumPre1 : Subsystem
  ChksumPre2 : Subsystem
  ChksumPre3 : Subsystem
  ChksumPre4 : Subsystem
  ChksumPre5 : Subsystem
  ChksumPre6 : Subsystem
  ChksumPre7 : Subsystem
  Constant : Constant  Value=256  OutDataTypeStr=uint16  SampleTime=-1
  Constant1 : Constant  Value=255  OutDataTypeStr=uint8  SampleTime=-1
  Constant2 : Constant  OutDataTypeStr=uint8  SampleTime=-1
  Constant3 : Constant  Value=0  OutDataTypeStr=uint8  SampleTime=-1
  Data Type Conversion6 : DataTypeConversion  OutDataTypeStr=uint8
  Math Function : Math  Operator=mod  OutputSignalType=real  SaturateOnIntegerOverflow=on
  Switch : Switch  Criteria=u2 ~= 0
  BOp_efChkSumErrFlg : Outport
  wires:
  Add2/1 -> Switch/2
  Add1/1 -> Add2/2
  Chksum in Frame/1 -> Add2/1
  ChksumPre3/1(Out1) -> Add/3
  ChksumPre2/1(Out1) -> Add/2
  Data Type Conversion6/1 -> Add1/2
  Add/1 -> Math Function/1
  Constant/1 -> Math Function/2
  Math Function/1 -> Data Type Conversion6/1
  Constant1/1 -> Add1/1
  BOp_bByte1/1 -> ChksumPre1/1(In1)
  ChksumPre1/1(Out1) -> Add/1
  BOp_bByte2/1 -> ChksumPre2/1(In1), ChksumPre3/1(In1), ChksumPre4/1(In1)
  ChksumPre4/1(Out1) -> Add/4
  BOp_bByte3/1 -> ChksumPre5/1(In1)
  BOp_bByte4/1 -> ChksumPre5/2(In2)
  ChksumPre5/1(Out1) -> Add/5
  BOp_bByte5/1 -> ChksumPre6/1(In1)
  BOp_bByte6/1 -> ChksumPre6/2(In2)
  ChksumPre6/1(Out1) -> Add/6
  ChksumPre7/1(Out1) -> Add/7
  BOp_bByte7/1 -> ChksumPre7/1(In1)
  Constant2/1 -> Switch/1
  Constant3/1 -> Switch/3
  Switch/1 -> BOp_efChkSumErrFlg/1

== system D53_LKA_Software/SignalBusCreator/Lanes Information Receive and Processing (LaneRx)/L1 Information (L1Info)/CAN Diagnosis (CANDia)/CheckSum Diagnosis (ChkSumDia)/Bit Check(BChk)/Bit Operating (BOp) ==
  note: CheckSum Error Flag Discription:
      | 1 : Fault
      | 0 : Normal
  note: Checksum Preprocess -- ChksumPre
  Chksum in Frame : Inport
  BOp_bByte1 : Inport  Port=2
  BOp_bByte2 : Inport  Port=3
  BOp_bByte3 : Inport  Port=4
  BOp_bByte4 : Inport  Port=5
  BOp_bByte5 : Inport  Port=6
  BOp_bByte6 : Inport  Port=7
  BOp_bByte7 : Inport  Port=8
  Add : Sum  Inputs=+++++++
  Add1 : Sum  Inputs=+-
  Add2 : Sum  Inputs=+-
  ChksumPre1 : Subsystem
  ChksumPre2 : Subsystem
  ChksumPre3 : Subsystem
  ChksumPre4 : Subsystem
  ChksumPre5 : Subsystem
  ChksumPre6 : Subsystem
  ChksumPre7 : Subsystem
  Constant : Constant  Value=256  OutDataTypeStr=uint16  SampleTime=-1
  Constant1 : Constant  Value=255  OutDataTypeStr=uint8  SampleTime=-1
  Constant2 : Constant  OutDataTypeStr=uint8  SampleTime=-1
  Constant3 : Constant  Value=0  OutDataTypeStr=uint8  SampleTime=-1
  Data Type Conversion6 : DataTypeConversion  OutDataTypeStr=uint8
  Math Function : Math  Operator=mod  OutputSignalType=real  SaturateOnIntegerOverflow=on
  Switch : Switch  Criteria=u2 ~= 0
  BOp_efChkSumErrFlg : Outport
  wires:
  Switch/1 -> BOp_efChkSumErrFlg/1
  Constant3/1 -> Switch/3
  Constant2/1 -> Switch/1
  BOp_bByte7/1 -> ChksumPre7/1(In1)
  ChksumPre7/1(Out1) -> Add/7
  ChksumPre6/1(Out1) -> Add/6
  BOp_bByte6/1 -> ChksumPre6/2(In2)
  BOp_bByte5/1 -> ChksumPre6/1(In1)
  ChksumPre5/1(Out1) -> Add/5
  BOp_bByte4/1 -> ChksumPre5/2(In2)
  BOp_bByte3/1 -> ChksumPre5/1(In1)
  ChksumPre4/1(Out1) -> Add/4
  BOp_bByte2/1 -> ChksumPre4/1(In1), ChksumPre3/1(In1), ChksumPre2/1(In1)
  ChksumPre1/1(Out1) -> Add/1
  BOp_bByte1/1 -> ChksumPre1/1(In1)
  Constant1/1 -> Add1/1
  Math Function/1 -> Data Type Conversion6/1
  Constant/1 -> Math Function/2
  Add/1 -> Math Function/1
  Data Type Conversion6/1 -> Add1/2
  ChksumPre2/1(Out1) -> Add/2
  ChksumPre3/1(Out1) -> Add/3
  Chksum in Frame/1 -> Add2/1
  Add1/1 -> Add2/2
  Add2/1 -> Switch/2

== system D53_LKA_Software/SignalBusCreator/Lanes Information Receive and Processing (LaneRx)/R0 Information (R0Info)/CAN Diagnosis (CANDia)/CheckSum Diagnosis (ChkSumDia)/Bit Check(BChk)/Bit Operating (BOp) ==
  note: CheckSum Error Flag Discription:
      | 1 : Fault
      | 0 : Normal
  note: Checksum Preprocess -- ChksumPre
  Chksum in Frame : Inport
  BOp_bByte1 : Inport  Port=2
  BOp_bByte2 : Inport  Port=3
  BOp_bByte3 : Inport  Port=4
  BOp_bByte4 : Inport  Port=5
  BOp_bByte5 : Inport  Port=6
  BOp_bByte6 : Inport  Port=7
  BOp_bByte7 : Inport  Port=8
  Add : Sum  Inputs=+++++++
  Add1 : Sum  Inputs=+-
  Add2 : Sum  Inputs=+-
  ChksumPre1 : Subsystem
  ChksumPre2 : Subsystem
  ChksumPre3 : Subsystem
  ChksumPre4 : Subsystem
  ChksumPre5 : Subsystem
  ChksumPre6 : Subsystem
  ChksumPre7 : Subsystem
  Constant : Constant  Value=256  OutDataTypeStr=uint16  SampleTime=-1
  Constant1 : Constant  Value=255  OutDataTypeStr=uint8  SampleTime=-1
  Constant2 : Constant  OutDataTypeStr=uint8  SampleTime=-1
  Constant3 : Constant  Value=0  OutDataTypeStr=uint8  SampleTime=-1
  Data Type Conversion6 : DataTypeConversion  OutDataTypeStr=uint8
  Math Function : Math  Operator=mod  OutputSignalType=real  SaturateOnIntegerOverflow=on
  Switch : Switch  Criteria=u2 ~= 0
  BOp_efChkSumErrFlg : Outport
  wires:
  Switch/1 -> BOp_efChkSumErrFlg/1
  Constant3/1 -> Switch/3
  Constant2/1 -> Switch/1
  BOp_bByte7/1 -> ChksumPre7/1(In1)
  ChksumPre7/1(Out1) -> Add/7
  ChksumPre6/1(Out1) -> Add/6
  BOp_bByte6/1 -> ChksumPre6/2(In2)
  BOp_bByte5/1 -> ChksumPre6/1(In1)
  ChksumPre5/1(Out1) -> Add/5
  BOp_bByte4/1 -> ChksumPre5/2(In2)
  BOp_bByte3/1 -> ChksumPre5/1(In1)
  ChksumPre4/1(Out1) -> Add/4
  BOp_bByte2/1 -> ChksumPre4/1(In1), ChksumPre3/1(In1), ChksumPre2/1(In1)
  ChksumPre1/1(Out1) -> Add/1
  BOp_bByte1/1 -> ChksumPre1/1(In1)
  Constant1/1 -> Add1/1
  Math Function/1 -> Data Type Conversion6/1
  Constant/1 -> Math Function/2
  Add/1 -> Math Function/1
  Data Type Conversion6/1 -> Add1/2
  ChksumPre2/1(Out1) -> Add/2
  ChksumPre3/1(Out1) -> Add/3
  Chksum in Frame/1 -> Add2/1
  Add1/1 -> Add2/2
  Add2/1 -> Switch/2

== system D53_LKA_Software/SignalBusCreator/Lanes Information Receive and Processing (LaneRx)/R1 Information (R1Info)/CAN Diagnosis (CANDia)/CheckSum Diagnosis (ChkSumDia)/Bit Check(BChk)/Bit Operating (BOp) ==
  note: Checksum Preprocess -- ChksumPre
  note: CheckSum Error Flag Discription:
      | 1 : Fault
      | 0 : Normal
  Chksum in Frame : Inport
  BOp_bByte1 : Inport  Port=2
  BOp_bByte2 : Inport  Port=3
  BOp_bByte3 : Inport  Port=4
  BOp_bByte4 : Inport  Port=5
  BOp_bByte5 : Inport  Port=6
  BOp_bByte6 : Inport  Port=7
  BOp_bByte7 : Inport  Port=8
  Add : Sum  Inputs=+++++++
  Add1 : Sum  Inputs=+-
  Add2 : Sum  Inputs=+-
  ChksumPre1 : Subsystem
  ChksumPre2 : Subsystem
  ChksumPre3 : Subsystem
  ChksumPre4 : Subsystem
  ChksumPre5 : Subsystem
  ChksumPre6 : Subsystem
  ChksumPre7 : Subsystem
  Constant : Constant  Value=256  OutDataTypeStr=uint16  SampleTime=-1
  Constant1 : Constant  Value=255  OutDataTypeStr=uint8  SampleTime=-1
  Constant2 : Constant  OutDataTypeStr=uint8  SampleTime=-1
  Constant3 : Constant  Value=0  OutDataTypeStr=uint8  SampleTime=-1
  Data Type Conversion6 : DataTypeConversion  OutDataTypeStr=uint8
  Math Function : Math  Operator=mod  OutputSignalType=real  SaturateOnIntegerOverflow=on
  Switch : Switch  Criteria=u2 ~= 0
  BOp_efChkSumErrFlg : Outport
  wires:
  Add2/1 -> Switch/2
  Add1/1 -> Add2/2
  Chksum in Frame/1 -> Add2/1
  ChksumPre3/1(Out1) -> Add/3
  ChksumPre2/1(Out1) -> Add/2
  Data Type Conversion6/1 -> Add1/2
  Add/1 -> Math Function/1
  Constant/1 -> Math Function/2
  Math Function/1 -> Data Type Conversion6/1
  Constant1/1 -> Add1/1
  BOp_bByte1/1 -> ChksumPre1/1(In1)
  ChksumPre1/1(Out1) -> Add/1
  BOp_bByte2/1 -> ChksumPre2/1(In1), ChksumPre3/1(In1), ChksumPre4/1(In1)
  ChksumPre4/1(Out1) -> Add/4
  BOp_bByte3/1 -> ChksumPre5/1(In1)
  BOp_bByte4/1 -> ChksumPre5/2(In2)
  ChksumPre5/1(Out1) -> Add/5
  BOp_bByte5/1 -> ChksumPre6/1(In1)
  BOp_bByte6/1 -> ChksumPre6/2(In2)
  ChksumPre6/1(Out1) -> Add/6
  ChksumPre7/1(Out1) -> Add/7
  BOp_bByte7/1 -> ChksumPre7/1(In1)
  Constant2/1 -> Switch/1
  Constant3/1 -> Switch/3
  Switch/1 -> BOp_efChkSumErrFlg/1

== system D53_LKA_Software/SignalBusCreator/Vehicle Movement Signal Receive and Processing (VehMovRx)/VehSpd CAN Frame PreProcess (VehSpdCANFrmPPrcs)/CAN Diagnosis (CANDia)/CheckSum Diagnosis (ChkSumDia)/Bit Check(BChk)/Bit Operating (BOp) ==
  note: CheckSum Error Flag Discription:
      | 1 : Fault
      | 0 : Normal
  note: Checksum Preprocess -- ChksumPre
  BOp_bByte0 : Inport
  BOp_bByte1 : Inport  Port=2
  BOp_bByte2 : Inport  Port=3
  BOp_bByte3 : Inport  Port=4
  BOp_bByte4 : Inport  Port=5
  BOp_bByte5 : Inport  Port=6
  BOp_bByte6 : Inport  Port=7
  BOp_bByte7 : Inport  Port=8
  Add : Sum  Inputs=+++++++
  Add1 : Sum  Inputs=+-
  Add2 : Sum  Inputs=+-
  ChksumPre1 : Subsystem
  ChksumPre2 : Subsystem
  ChksumPre3 : Subsystem
  ChksumPre4 : Subsystem
  ChksumPre5 : Subsystem
  ChksumPre6 : Subsystem
  ChksumPre7 : Subsystem
  Constant : Constant  Value=256  OutDataTypeStr=uint16  SampleTime=-1
  Constant1 : Constant  Value=255  OutDataTypeStr=uint8  SampleTime=-1
  Constant2 : Constant  OutDataTypeStr=uint8  SampleTime=-1
  Constant3 : Constant  Value=0  OutDataTypeStr=uint8  SampleTime=-1
  Data Type Conversion6 : DataTypeConversion  OutDataTypeStr=uint8
  Math Function : Math  Operator=mod  OutputSignalType=real  SaturateOnIntegerOverflow=on
  Switch : Switch  Criteria=u2 ~= 0
  BOp_efChkSumErrFlg : Outport
  wires:
  Switch/1 -> BOp_efChkSumErrFlg/1
  Constant3/1 -> Switch/3
  Constant2/1 -> Switch/1
  BOp_bByte7/1 -> ChksumPre7/1(In1)
  ChksumPre7/1(Out1) -> Add/7
  ChksumPre6/1(Out1) -> Add/6
  BOp_bByte6/1 -> ChksumPre6/2(In2)
  BOp_bByte5/1 -> ChksumPre6/1(In1)
  ChksumPre5/1(Out1) -> Add/5
  BOp_bByte4/1 -> ChksumPre5/2(In2)
  BOp_bByte3/1 -> ChksumPre5/1(In1)
  ChksumPre4/1(Out1) -> Add/4
  BOp_bByte2/1 -> ChksumPre4/1(In1), ChksumPre3/1(In1), ChksumPre2/1(In1)
  ChksumPre1/1(Out1) -> Add/1
  BOp_bByte1/1 -> ChksumPre1/1(In1)
  Constant1/1 -> Add1/1
  Math Function/1 -> Data Type Conversion6/1
  Constant/1 -> Math Function/2
  Add/1 -> Math Function/1
  Data Type Conversion6/1 -> Add1/2
  ChksumPre2/1(Out1) -> Add/2
  ChksumPre3/1(Out1) -> Add/3
  BOp_bByte0/1 -> Add2/1
  Add1/1 -> Add2/2
  Add2/1 -> Switch/2

== system D53_LKA_Software/SignalBusCreator/Vehicle Movement Signal Receive and Processing (VehMovRx)/Yaw State CAN Frame PreProcess (YawCANFrmPPrcs)/CAN Diagnosis (CANDia)/CheckSum Diagnosis (ChkSumDia)/Bit Check(BChk)/Bit Operating (BOp) ==
  note: CheckSum Error Flag Discription:
      | 1 : Fault
      | 0 : Normal
  note: Checksum Preprocess -- ChksumPre
  BOp_bByte0 : Inport
  BOp_bByte1 : Inport  Port=2
  BOp_bByte2 : Inport  Port=3
  BOp_bByte3 : Inport  Port=4
  BOp_bByte4 : Inport  Port=5
  BOp_bByte5 : Inport  Port=6
  BOp_bByte6 : Inport  Port=7
  BOp_bByte7 : Inport  Port=8
  Add : Sum  Inputs=+++++++
  Add1 : Sum  Inputs=+-
  Add2 : Sum  Inputs=+-
  ChksumPre1 : Subsystem
  ChksumPre2 : Subsystem
  ChksumPre3 : Subsystem
  ChksumPre4 : Subsystem
  ChksumPre5 : Subsystem
  ChksumPre6 : Subsystem
  ChksumPre7 : Subsystem
  Constant : Constant  Value=256  OutDataTypeStr=uint16  SampleTime=-1
  Constant1 : Constant  Value=255  OutDataTypeStr=uint8  SampleTime=-1
  Constant2 : Constant  OutDataTypeStr=uint8  SampleTime=-1
  Constant3 : Constant  Value=0  OutDataTypeStr=uint8  SampleTime=-1
  Data Type Conversion6 : DataTypeConversion  OutDataTypeStr=uint8
  Math Function : Math  Operator=mod  OutputSignalType=real  SaturateOnIntegerOverflow=on
  Switch : Switch  Criteria=u2 ~= 0
  BOp_efChkSumErrFlg : Outport
  wires:
  Switch/1 -> BOp_efChkSumErrFlg/1
  Constant3/1 -> Switch/3
  Constant2/1 -> Switch/1
  BOp_bByte7/1 -> ChksumPre7/1(In1)
  ChksumPre7/1(Out1) -> Add/7
  ChksumPre6/1(Out1) -> Add/6
  BOp_bByte6/1 -> ChksumPre6/2(In2)
  BOp_bByte5/1 -> ChksumPre6/1(In1)
  ChksumPre5/1(Out1) -> Add/5
  BOp_bByte4/1 -> ChksumPre5/2(In2)
  BOp_bByte3/1 -> ChksumPre5/1(In1)
  ChksumPre4/1(Out1) -> Add/4
  BOp_bByte2/1 -> ChksumPre4/1(In1), ChksumPre3/1(In1), ChksumPre2/1(In1)
  ChksumPre1/1(Out1) -> Add/1
  BOp_bByte1/1 -> ChksumPre1/1(In1)
  Constant1/1 -> Add1/1
  Math Function/1 -> Data Type Conversion6/1
  Constant/1 -> Math Function/2
  Add/1 -> Math Function/1
  Data Type Conversion6/1 -> Add1/2
  ChksumPre2/1(Out1) -> Add/2
  ChksumPre3/1(Out1) -> Add/3
  BOp_bByte0/1 -> Add2/1
  Add1/1 -> Add2/2
  Add2/1 -> Switch/2

== system D53_LKA_Software/LL/LLOn/LKA/LKA Motion Planning (LKAMP) /Switching Condition (SwtCon)/Ending Heading Angle Determination (EndHdAgDet)/Lateral Speed Compensation (LSpdComp)/If Action Subsystem ==
  In1 : Inport
  Action Port : ActionPort  InitializeStates=reset
  Cast To Single1 : DataTypeConversion  LockScale=on
  Out1 : Outport  InitialOutput=0
  wires:
  Cast To Single1/1 -> Out1/1
  In1/1 -> Cast To Single1/1

== system D53_LKA_Software/LL/LLOn/LKA/LKA Motion Planning (LKAMP) /Switching Condition (SwtCon)/Ending Heading Angle Determination (EndHdAgDet)/Lateral Speed Compensation (LSpdComp)/If Action Subsystem2 ==
  Action Port : ActionPort  InitializeStates=reset
  Constant : Constant  Value=0  OutDataTypeStr=single
  Out1 : Outport  InitialOutput=0
  wires:
  Constant/1 -> Out1/1

== system D53_LKA_Software/LL/LLOn/LKA/LKA Motion Planning (LKAMP) /Switching Condition (SwtCon)/Ending Heading Angle Determination (EndHdAgDet)/Lateral Speed Compensation (LSpdComp)/If Action Subsystem4 ==
  In1 : Inport
  Action Port : ActionPort  InitializeStates=reset
  Cast To Single1 : DataTypeConversion  LockScale=on
  Out1 : Outport  InitialOutput=0
  wires:
  Cast To Single1/1 -> Out1/1
  In1/1 -> Cast To Single1/1

== system D53_LKA_Software/LL/LLOn/LKA/Lane Following (LF)/Trajectory Following Control (TFC)/Feedback Control (FbCtl)/Subsystem/If Action Subsystem ==
  In1 : Inport
  Action Port : ActionPort
  Out1 : Outport
  wires:
  In1/1 -> Out1/1

== system D53_LKA_Software/LL/LLOn/LKA/Lane Following (LF)/Trajectory Following Control (TFC)/Feedback Control (FbCtl)/Subsystem/If Action Subsystem1 ==
  In1 : Inport
  Action Port : ActionPort
  Out1 : Outport
  wires:
  In1/1 -> Out1/1

== system D53_LKA_Software/LL/LLOn/LKA/Lane Following (LF)/Trajectory Following Control (TFC)/Feedback Control (FbCtl)/Subsystem/If Action Subsystem2 ==
  In1 : Inport
  Action Port : ActionPort
  Out1 : Outport
  wires:
  In1/1 -> Out1/1

== system D53_LKA_Software/LL/LLOn/LKA/Lane Following (LF)/Trajectory Following Control (TFC)/Feedback Control (FbCtl)/Subsystem/Signal Latching2 ==
  In : Inport
  Add : Sum  OutDataTypeStr=uint16
  Constant : Constant  OutDataTypeStr=uint16  SampleTime=-1
  Constant2 : Constant  Value=LatchTime  OutDataTypeStr=uint16  SampleTime=-1
  If : If  NumInputs=2  IfExpression=u1==u2  ShowElse=off
  Memory : Memory  InheritSampleTime=on
  Saturation1 : Saturate  UpperLimit=10000  LowerLimit=0  OutDataTypeStr=uint16
  "if action " : Subsystem  TreatAsAtomicUnit=on
  Out : Outport
  wires:
  Constant2/1 -> If/2
  In/1 -> "if action "/1(In)
  "if action "/1(Out) -> Out/1
  If/1 -> "if action "/Action
  Constant/1 -> Add/1
  Add/1 -> Saturation1/1
  Memory/1 -> Add/2
  Saturation1/1 -> Memory/1, If/1

== system D53_LKA_Software/LL/LLOn/LKA/Plan To LaneFollowing (PTLF)/InsideJudge1/If Action Subsystem/If Action Subsystem/Signal Latching ==
  In : Inport
  Add : Sum  OutDataTypeStr=uint16
  Constant : Constant  OutDataTypeStr=uint16  SampleTime=-1
  Constant2 : Constant  Value=LatchTime  OutDataTypeStr=uint16  SampleTime=-1
  If : If  NumInputs=2  IfExpression=u1<=u2  ShowElse=off
  Memory : Memory  InheritSampleTime=on
  Saturation1 : Saturate  UpperLimit=10000  LowerLimit=0  OutDataTypeStr=uint16
  "if action " : Subsystem  TreatAsAtomicUnit=on
  Out : Outport
  wires:
  Saturation1/1 -> If/1, Memory/1
  Memory/1 -> Add/2
  Add/1 -> Saturation1/1
  Constant/1 -> Add/1
  If/1 -> "if action "/Action
  "if action "/1(Out) -> Out/1
  In/1 -> "if action "/1(In)
  Constant2/1 -> If/2
